simulink model "Albo_JL_MATLAB_No6"  (R2023b)
settings: Solver=VariableStepAuto  StartTime=0.0  StopTime=10.0  RelTol=1e-3
settings Model: Creator=ACER  LastModifiedBy=ACER

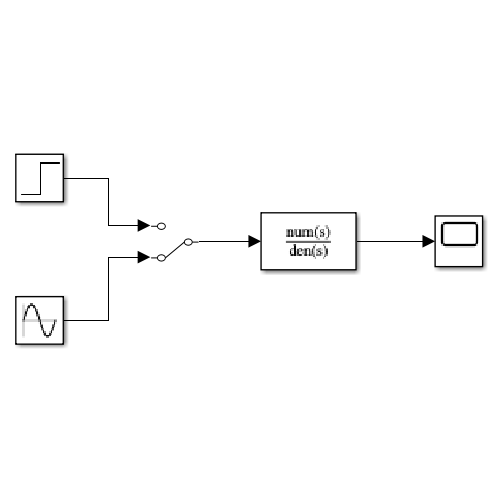
[thumbnail: Simulink's stored preview of the top-level diagram]
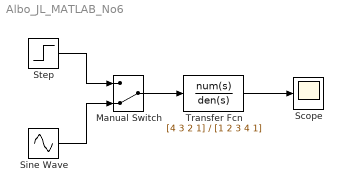
== system Albo_JL_MATLAB_No6 ==
  Manual Switch : ManualSwitch  CurrentSetting=0
  Scope : Scope
  Sine Wave : Sin  SampleTime=0
  Step : Step  Time=0  SampleTime=0
  Transfer Fcn : TransferFcn  Numerator=[4 3 2 1]  Denominator=[1 2 3 4 1]
  wires:
  Transfer Fcn/1 -> Scope/1
  Sine Wave/1 -> Manual Switch/2
  Step/1 -> Manual Switch/1
  Manual Switch/1 -> Transfer Fcn/1
